simulink model "falling_ball_sim"  (R2020a)
settings: Solver=FixedStepDiscrete  StartTime=0.0  StopTime=10.0  FixedStep=.01  RelTol=1e-3
values from neighbouring files (symbols this model uses):
  Cd = 0.47    [parameters.m]
  g = 9.81    [parameters.m]
  G = 6.674e-11    [parameters.m]
  m = 0.100    (= 0.1)    [parameters.m]
  M = 5.972e24    (= 5.972e+24)    [parameters.m]
  r = 0.05    [parameters.m]
  R = 6371e3    (= 6371000)    [parameters.m]
  rho = 1.293    [parameters.m]
undefined symbols (not defined in the file or in its folder): DiscIntNeverNeededParam, init
settings Model: Creator=AC45903  LastModifiedBy=AC45903

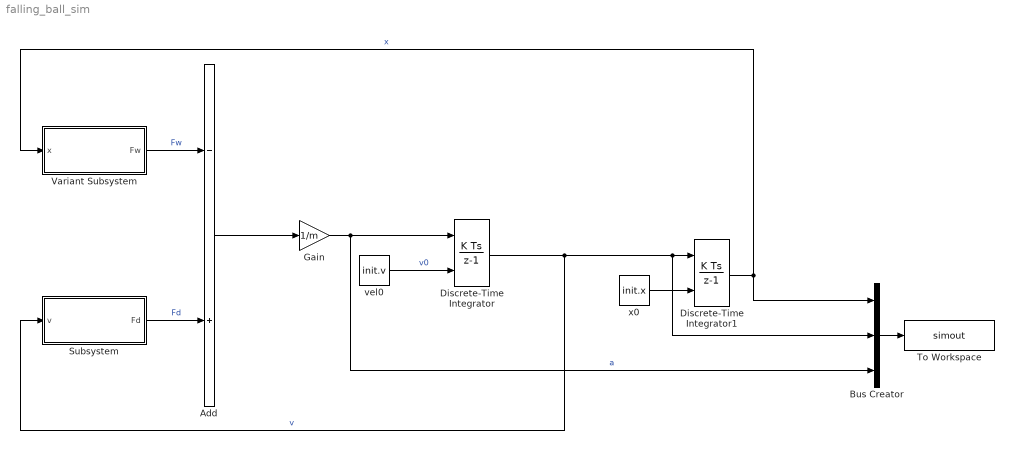
== system falling_ball_sim ==
  Add : Sum  Inputs=-+
  Bus Creator : BusCreator  Inputs=3
  Discrete-Time Integrator : DiscreteIntegrator  InitialConditionSource=external  SampleTime=-1  ICPrevOutput=DiscIntNeverNeededParam  ICPrevScaledInput=DiscIntNeverNeededParam
  Discrete-Time Integrator1 : DiscreteIntegrator  InitialConditionSource=external  SampleTime=-1  ICPrevOutput=DiscIntNeverNeededParam  ICPrevScaledInput=DiscIntNeverNeededParam
  Gain : Gain  Gain=1/m
  Subsystem : Subsystem
  To Workspace : ToWorkspace  VariableName=simout  SaveFormat=Timeseries  SampleTime=-1
  Variant Subsystem : Subsystem  Variant=on
  vel0 : Constant  Value=init.v
  x0 : Constant  Value=init.x
  wires:
  Add/1 -> Gain/1
  vel0/1 -> Discrete-Time Integrator/2  "v0"
  Gain/1 -> Bus Creator/3, Discrete-Time Integrator/1  "a"
  Discrete-Time Integrator/1 -> Subsystem/1(v), Bus Creator/2, Discrete-Time Integrator1/1  "v"
  x0/1 -> Discrete-Time Integrator1/2
  Discrete-Time Integrator1/1 -> Variant Subsystem/1(x), Bus Creator/1  "x"
  Variant Subsystem/1(Fw) -> Add/1  "Fw"
  Subsystem/1(Fd) -> Add/2  "Fd"
  Bus Creator/1 -> To Workspace/1

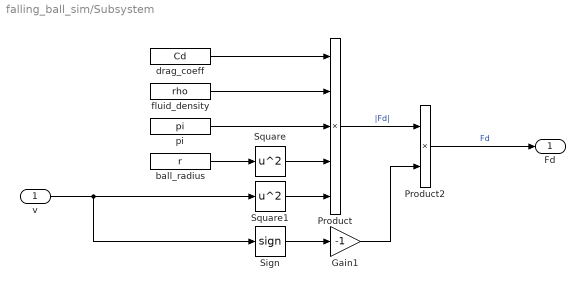
== system falling_ball_sim/Subsystem ==
  v : Inport
  Gain1 : Gain  Gain=-1
  Product : Product  Inputs=5
  Product2 : Product
  Sign : Signum
  Square : Math  Operator=square  SaturateOnIntegerOverflow=on
  Square1 : Math  Operator=square  SaturateOnIntegerOverflow=on
  ball_radius : Constant  Value=r
  drag_coeff : Constant  Value=Cd
  fluid_density : Constant  Value=rho
  pi : Constant  Value=pi
  Fd : Outport
  wires:
  pi/1 -> Product/3
  v/1 -> Sign/1, Square1/1
  Sign/1 -> Gain1/1
  Gain1/1 -> Product2/2
  fluid_density/1 -> Product/2
  ball_radius/1 -> Square/1
  drag_coeff/1 -> Product/1
  Square/1 -> Product/4
  Product/1 -> Product2/1  "|Fd|"
  Square1/1 -> Product/5
  Product2/1 -> Fd/1  "Fd"

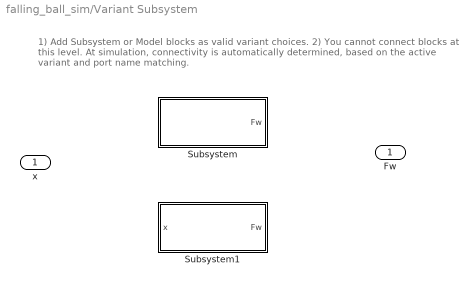
== system falling_ball_sim/Variant Subsystem ==
  note: 1) Add Subsystem or Model blocks as valid variant choices.
      | 2) You cannot connect blocks at this level. At simulation, connectivity is automatically
      | determined, based on the active variant and port name matching.
  x : Inport
  Subsystem : Subsystem  VariantControl=gravity_law==0
  Subsystem1 : Subsystem  VariantControl=gravity_law==1
  Fw : Outport

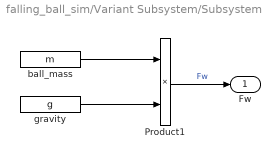
== system falling_ball_sim/Variant Subsystem/Subsystem ==
  Product1 : Product
  ball_mass : Constant  Value=m
  gravity : Constant  Value=g
  Fw : Outport
  wires:
  ball_mass/1 -> Product1/1
  gravity/1 -> Product1/2
  Product1/1 -> Fw/1  "Fw"

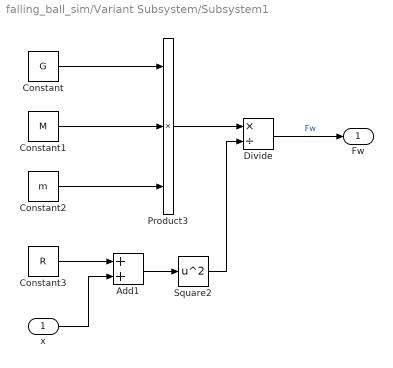
== system falling_ball_sim/Variant Subsystem/Subsystem1 ==
  x : Inport
  Add1 : Sum
  Constant : Constant  Value=G
  Constant1 : Constant  Value=M
  Constant2 : Constant  Value=m
  Constant3 : Constant  Value=R
  Divide : Product  Inputs=*/
  Product3 : Product  Inputs=3
  Square2 : Math  Operator=square  SaturateOnIntegerOverflow=on
  Fw : Outport
  wires:
  Square2/1 -> Divide/2
  Constant2/1 -> Product3/3
  Divide/1 -> Fw/1  "Fw"
  Constant3/1 -> Add1/1
  x/1 -> Add1/2
  Product3/1 -> Divide/1
  Constant1/1 -> Product3/2
  Add1/1 -> Square2/1
  Constant/1 -> Product3/1
